simulink model "carro"  (Simulink 7.0)
settings: Solver=ode45  StartTime=0.0  StopTime=10.0  RelTol=1e-3
values from neighbouring files (symbols this model uses):
  b = 0.1    [consCarroMasa.m]
  k = 10    [consCarroMasa.m]
  m = 1    [consCarroMasa.m]
settings Model: Creator=Usuario  LastModifiedBy=Usuario

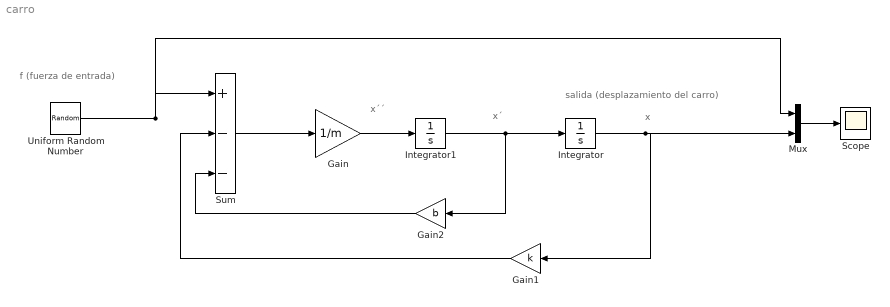
== system carro ==
  note: x´
  note: x
  note: x´´
  note: f (fuerza de entrada)
  note: salida (desplazamiento del carro)
  Gain : Gain  Gain=1/m  ParameterDataType=sfix(16)  ParameterScaling=2^0  OutDataType=sfix(16)  OutScaling=2^0
  Gain1 : Gain  Orientation=left  Gain=k  ParameterDataType=sfix(16)  ParameterScaling=2^0  OutDataType=sfix(16)  OutScaling=2^0
  Gain2 : Gain  Orientation=left  Gain=b  ParameterDataType=sfix(16)  ParameterScaling=2^0  OutDataType=sfix(16)  OutScaling=2^0
  Integrator : Integrator
  Integrator1 : Integrator
  Mux : Mux  Inputs=2
  Scope : Scope
  Sum : Sum  Inputs=|+--  OutDataType=sfix(16)  OutScaling=2^0
  Uniform Random Number : UniformRandomNumber  SampleTime=1
  wires:
  Integrator1/1 -> Integrator/1, Gain2/1
  Gain/1 -> Integrator1/1
  Sum/1 -> Gain/1
  Integrator/1 -> Gain1/1, Mux/2
  Gain1/1 -> Sum/2
  Gain2/1 -> Sum/3
  Uniform Random Number/1 -> Sum/1, Mux/1
  Mux/1 -> Scope/1
